simulink model "untitled5"  (R2025a)
settings: Solver=VariableStepAuto  StartTime=0.0  StopTime=10.0  RelTol=1e-3
libraries: fuzblock x1
settings Model: Creator=Win 11  LastModifiedBy=Win 11

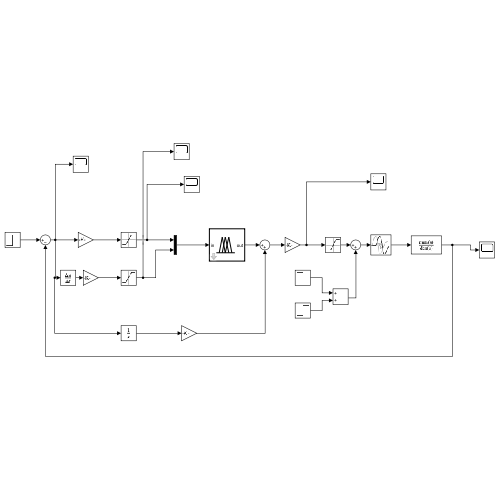
[thumbnail: Simulink's stored preview of the top-level diagram]
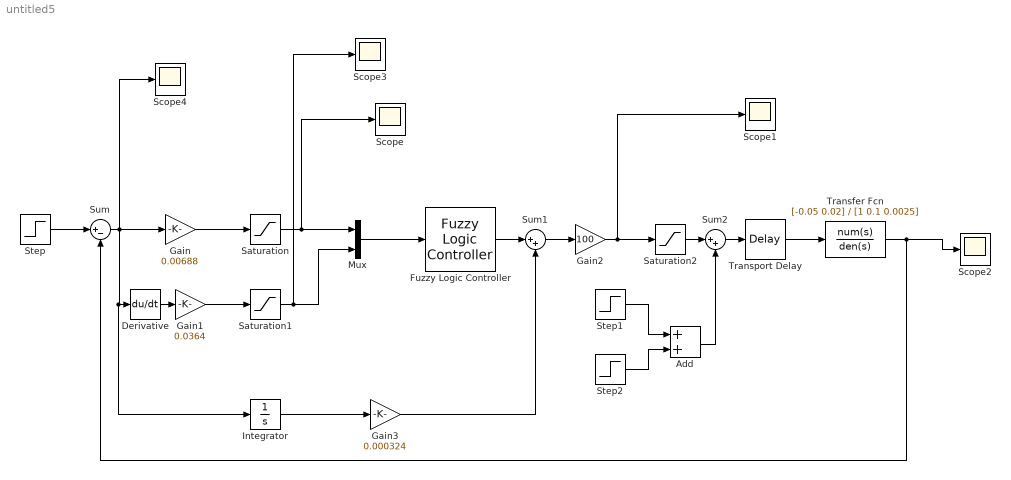
== system untitled5 ==
  Add : Sum
  Derivative : Derivative
  Fuzzy Logic Controller : fuzblock/Fuzzy Logic  Controller  FIS=fis  OutputSampleNumber=101  DataType=double  UseLookupTable=off  NumBreakpoints=10  FuzzifiedInputs=off  RuleFiringStrengths=off  RuleOutputs=off  AggregatedOutputs=off  SimulateUsing=Interpreted execution  OutOfRangeInputValueMessage=warning  NoRuleFiredMessage=warning  EmptyOutputFuzzySetMessage=warning
  Gain : Gain  Gain=0.00688
  Gain1 : Gain  Gain=0.0364
  Gain2 : Gain  Gain=100
  Gain3 : Gain  Gain=0.000324
  Integrator : Integrator
  Mux : Mux  Inputs=2
  Saturation : Saturate  UpperLimit=4  LowerLimit=-4
  Saturation1 : Saturate  UpperLimit=4  LowerLimit=-4
  Saturation2 : Saturate  UpperLimit=+2.2  LowerLimit=-2.2
  Scope{,1..4} (5 alike) : Scope
      Scope settings: ActiveDisplayYMinimum=-0.0012909040384079347  ActiveDisplayYMaximum=0.003432922309414564
      Scope1 settings: ActiveDisplayYMinimum=-0.15265048126211622  ActiveDisplayYMaximum=0.27286049111293736
      Scope2 settings: ActiveDisplayYMinimum=-0.49897126590327967  ActiveDisplayYMaximum=0.18763140093138586  DataLoggingVariableName=ScopeData2
      Scope3 settings: ActiveDisplayYMinimum=-0.0053158739968185128  ActiveDisplayYMaximum=0.0078105479592406142  DataLoggingVariableName=ScopeData3
      Scope4 settings: ActiveDisplayYMinimum=-0.18763140093138586  ActiveDisplayYMaximum=0.49897126590327967  DataLoggingVariableName=ScopeData4
  Step : Step  After=0  SampleTime=0
  Step1 : Step  After=-2.2  SampleTime=0
  Step2 : Step  Time=5  After=2.2  SampleTime=0
  Sum : Sum  Inputs=|+-
  Sum1 : Sum  Inputs=|++
  Sum2 : Sum  Inputs=|++
  Transfer Fcn : TransferFcn  Numerator=[-0.05 0.02]  Denominator=[1 0.1 0.0025]
  Transport Delay : TransportDelay  DelayTime=2
  wires:
  Step/1 -> Sum/1
  Gain/1 -> Saturation/1
  Saturation/1 -> Scope/1, Mux/1
  Saturation1/1 -> Scope3/1, Mux/2
  Mux/1 -> Fuzzy Logic Controller/1
  Fuzzy Logic Controller/1 -> Sum1/1
  Sum1/1 -> Gain2/1
  Gain2/1 -> Scope1/1, Saturation2/1
  Transport Delay/1 -> Transfer Fcn/1
  Transfer Fcn/1 -> Scope2/1, Sum/2
  Integrator/1 -> Gain3/1
  Gain3/1 -> Sum1/2
  Gain1/1 -> Saturation1/1
  Derivative/1 -> Gain1/1
  Sum/1 -> Scope4/1, Gain/1, Integrator/1, Derivative/1
  Saturation2/1 -> Sum2/1
  Sum2/1 -> Transport Delay/1
  Add/1 -> Sum2/2
  Step1/1 -> Add/1
  Step2/1 -> Add/2
